simulink subsystem "Body2World"  (R2024a)
settings: Solver=VariableStepAuto  StartTime=0.0  StopTime=10.0  RelTol=1e-3
model mask{InitialCondition=eta_Init}
  mask prompts: InitialCondition "Simulink:blkprm_prompts:IntegratorInitCond"
settings Model: Creator=esben  LastModifiedBy=BP21JL
settings SolverCC: AlgebraicLoopSolver=TrustRegion
settings DebuggingCC: UnconnectedInputMsg=warning  UnconnectedOutputMsg=warning  UnconnectedLineMsg=warning
settings ModelReferenceCC: EnableRefExpFcnMdlSchedulingChecks=on
settings RTWCC: GPUComputeCapability=3.5

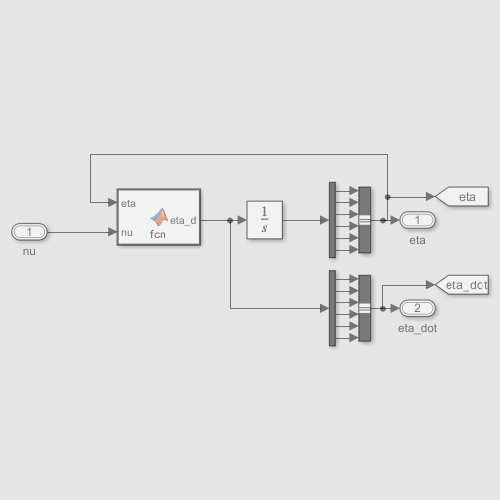
[thumbnail: Simulink's stored preview of the top-level diagram]
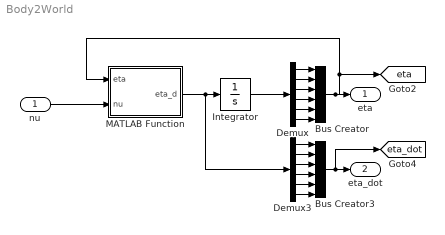
== system Body2World ==
  nu : Inport  OutDataTypeStr=Bus: nu
  Bus Creator : BusCreator  Inputs=6  OutDataTypeStr=Bus: eta
      settings: InheritFromInputs=off
  Bus Creator3 : BusCreator  Inputs=6  OutDataTypeStr=Bus: eta_d
      settings: InheritFromInputs=off
  Demux : Demux  Outputs=6
  Demux3 : Demux  Outputs=6
  Integrator : Integrator  InitialCondition=InitialCondition
  MATLAB Function : MATLAB Function  TreatAsAtomicUnit=on
  eta : Outport  OutDataTypeStr=Bus: eta
  eta_dot : Outport  Port=2  OutDataTypeStr=Bus: eta_d
  tag scope: eta=global, eta_dot=global
  wires:
  Demux3/3 -> Bus Creator3/3
  MATLAB Function/1(eta_d) -> Integrator/1, Demux3/1
  Demux3/4 -> Bus Creator3/4
  Demux/4 -> Bus Creator/4
  Demux/5 -> Bus Creator/5
  Demux/1 -> Bus Creator/1
  Integrator/1 -> Demux/1
  Demux/3 -> Bus Creator/3
  Demux3/1 -> Bus Creator3/1
  Demux3/6 -> Bus Creator3/6
  Demux/6 -> Bus Creator/6
  Demux3/2 -> Bus Creator3/2
  Demux/2 -> Bus Creator/2
  Demux3/5 -> Bus Creator3/5
  Bus Creator/1 -> eta/1, MATLAB Function/1(eta), [eta]
  Bus Creator3/1 -> eta_dot/1, [eta_dot]
  nu/1 -> MATLAB Function/2(nu)

== matlab function Body2World/MATLAB Function ==
  data: eta input Bus: eta; nu input Bus: nu; eta_d output
function eta_d = fcn(eta,nu)

eta_d = [Rotn_b(eta.phi,eta.theta,eta.psi) zeros(3,3);zeros(3,3) TransAng(eta.phi,eta.theta,eta.psi)]*struct2vec(nu);
